simulink model "Model_1"  (R2020b)
settings: Solver=VariableStepAuto  StartTime=0.0  StopTime=100.0  RelTol=1e-3
values from neighbouring files (symbols this model uses):
  b = 50    [Script1.m]
  k1 = 50    [Script1.m]
  k2 = 25    [Script1.m]
  m1 = 100    [Script1.m]
  m2 = 20    [Script1.m]
settings Model: Creator=Diwakar Reddy  LastModifiedBy=Diwakar Reddy

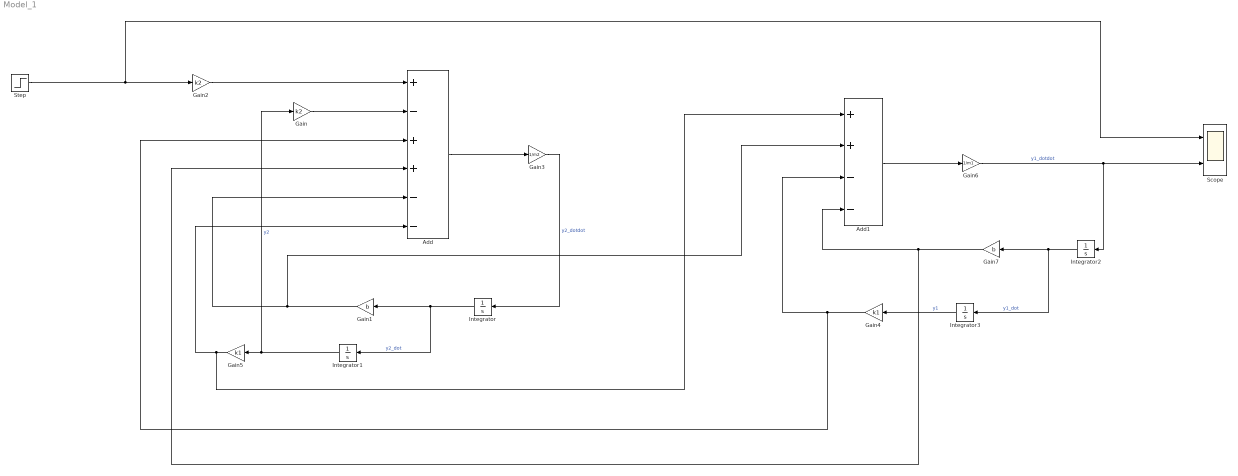
== system Model_1 ==
  Add : Sum  Inputs=+-++--
  Add1 : Sum  Inputs=++--
  Gain : Gain  Gain=k2
  Gain1 : Gain  Gain=b
  Gain2 : Gain  Gain=k2
  Gain3 : Gain  Gain=1/m2
  Gain4 : Gain  Gain=k1
  Gain5 : Gain  Gain=k1
  Gain6 : Gain  Gain=1/m1
  Gain7 : Gain  Gain=b
  Integrator{,1..3} (4 alike) : Integrator
  Scope : Scope  NumInputPorts=2
  Step : Step  SampleTime=0
  wires:
  Add/1 -> Gain3/1
  Gain2/1 -> Add/1
  Step/1 -> Scope/1, Gain2/1
  Gain4/1 -> Add/3, Add1/3
  Gain3/1 -> Integrator/1  "y2_dotdot"
  Integrator/1 -> Integrator1/1, Gain1/1  "y2_dot"
  Gain1/1 -> Add1/2, Add/5
  Integrator1/1 -> Gain/1, Gain5/1  "y2"
  Gain5/1 -> Add/6, Add1/1
  Add1/1 -> Gain6/1
  Gain6/1 -> Integrator2/1, Scope/2  "y1_dotdot"
  Integrator2/1 -> Integrator3/1, Gain7/1  "y1_dot"
  Gain7/1 -> Add1/4, Add/4
  Integrator3/1 -> Gain4/1  "y1"
  Gain/1 -> Add/2
